simulink model "Horizontal_Turn_Symmetric_DOP"  (Simulink 9.2)
settings: Solver=ode4  StartTime=0.0  StopTime=50  FixedStep=0.01  RelTol=1e-1
values from neighbouring files (symbols this model uses):
  alpha_ = atan(y(3)/y(1))    [Trim_sym.m]    (also in Trim_sym.mat = 0.357010867724)
  b = 2.8956    [Constants_sym.m]    (also in Trim_sym_main.m)
  cbar = 0.18994    [Constants_sym.m]    (also in Trim_sym_main.m)
  Cprop = 1    [Constants_sym.m]    (also in Trim_sym_main.m)
  d2r = pi/180    (= 0.0174532925199)    [Constants_sym.m]    (also in Trim_sym.m; Trim_sym_main.m)
  g = 9.81    [Constants_sym.m]    (also in Trim_sym_main.m)
  Ixx = 0.8244    [Constants_sym.m]    (also in Trim_sym_main.m)
  Ixz = 0.1204    [Constants_sym.m]    (also in Trim_sym_main.m)
  Iyy = 1.135    [Constants_sym.m]    (also in Trim_sym_main.m)
  Izz = 1.759    [Constants_sym.m]    (also in Trim_sym_main.m)
  Kmotor = 80    [Constants_sym.m]    (also in Trim_sym_main.m)
  m = 13.5    [Constants_sym.m]    (also in Trim_sym_main.m)
  q = 0    [Trim_sym.m]
  qbar = 0.5*rho*V^2    [Constants_sym.m]    (also in Trim_sym_main.m = 186.625322459)
  r = 0    [Trim_sym.m]
  r2d = 180/pi    (= 57.2957795131)    [Constants_sym.m]    (also in Trim_sym.m; Trim_sym_main.m)
  rho = p_atm/(287*T_atm)    [Constants_sym.m]    (also in Trim_sym_main.m = 1.44533597728)
  S = 0.55    [Constants_sym.m]    (also in Trim_sym_main.m)
  Sprop = 0.2027    [Constants_sym.m]    (also in Trim_sym_main.m)
  V = 16.07    [Trim_sym.mat]    (also in Trim_sym_main.m)
undefined symbols (not defined in the file or in its folder): F, Light, MIL, sigbuilder_block
libraries: simulink x4, aerolibwind2 x3, sharedtransform x1
(part 2 of 2)

== matlab function EOM/Aerodynamic Constants 2 ==
  data: alpha_ input double; Cx output double; beta_ input double; P input double; Q input double; R input double; delA input double; delE input double; delR input double; Cy output double; Cz output double; Cl output double; Cm output double; Cn output double; u input double; v input double; w input double; CD output double; CL output double
function [Cx,Cy,Cz,Cl,Cm,Cn,CD, CL] = Constants(alpha_,beta_,P,Q,R,delA,delE,delR,u,v,w)

d2r = pi/180;
r2d = 180/pi;

%% CONSTANTS
% Geometric / mass properties data
g = 9.81; 
ALT = 1000; % altitude (in m)
V = sqrt(u^2 + v^2 + w^2); % velocity (in m/s)

% max_thrust = 32000*g/2.2046;
if (ALT <= 11000) 
   T_atm = 288.15-0.0065*ALT; % atmospheric temp.(in Kelvin)
   p_atm = 101325*(T_atm/288.15)^(9.81/(287*0.0065));  % atmospheric pressure (pascal)
else 
   T_atm = 216.65;
   p_atm = 22632*exp(-9.81*(ALT-11000)/(287*216.65)); 
end   
R1 = 287.1;  % Gas constant (m2/s2/K)
ss = sqrt(1.4*R1*T_atm); % sound velocity (m/s)
M = V/ss;
rho = p_atm/(287*T_atm);
rho_sl = 1.225; % density @ sea-level (kg/m3)
% T = max_thrust * (rho / rho_sl)^0.7 * (1 - exp((ALT - 17000) / 2000));
% T = 0.9*max_thrust*(0.88+0.24*(abs(M-0.6))^1.4)*(rho/rho_sl)^0.8;

lz = 0;
lx = 0;
 m = 13.5;
 W = m*g;
 S = 0.55;
 qbar = 0.5*rho*V^2;
 cbar = 0.18994;
b = 2.8956; % ft -> m  
 Ixx = 0.8244; % slugs ft2 -> Kg m2
Iyy = 1.135;
Izz = 1.759;
Ixz = 0.1204;

%%

CD0 = 0.03;
CDalpha = 0.30;
CDQ=0;
CDdeltae=0;
CDP=0.0437;
CD = (CD0+CDalpha*alpha_+(CDQ*cbar*Q/(2*V))+CDdeltae*delE+(CDP*b*P/(2*V)));
 
CY0=0;
CYbeta = -0.98;
CYP = 0;
CYR = 0;
CYdeltaa = 0;
CYdeltar = -0.17;

CY = (CY0+CYbeta*beta_+(CYP*b*P/(2*V))+(CYR*b*R/(2*V))+CYdeltaa*delA+CYdeltar*delR);
 
CL0=0.28;
CLalpha = 3.45;
CLQ=0;
CLdeltae = -0.36;
CL = (CL0 + CLalpha*alpha_+CLdeltae*delE+(CLQ*cbar*Q/(2*V)));
 
CM0 = -0.02338;
CMalpha = -0.38;
CMQ = -3.6;
CMdeltae = -0.5;
Cm = (CM0+CMalpha*alpha_+CMdeltae*delE+(CMQ*cbar*Q/(2*V)));
 
Cl0=0;
Clbeta =-0.12;
ClP = -0.26;
ClR = 0.14;
Cldeltaa = 0.08;
Cldeltar = 0.105;

Cl = (Cl0+Clbeta*beta_+(ClP*b*P/(2*V))+(ClR*b*R/(2*V))+Cldeltaa*delA+ Cldeltar*delR);
 
Cn0=0;
Cnbeta = 0.25;
CnP = 0.022;
CnR = -0.35;
Cndeltaa = 0.06;
Cndeltar = -0.032;
Cn = (Cn0+Cnbeta*beta_+(CnP*b*P/(2*V))+(CnR*b*R/(2*V))+Cndeltaa*delA+Cndeltar*delR);
 
Cx = (-CD*cos(alpha_)*cos(beta_)-CY*cos(alpha_)*sin(beta_)+CL*sin(alpha_));
Cy = (CY*cos(beta_)-CD*sin(beta_));
Cz = (-CD*sin(alpha_)*cos(beta_)-CY*sin(alpha_)*sin(beta_)-CL*cos(alpha_));

== matlab function Lateral Directional Controller (backstepping)/Back_Step ==
  data: alpha_ input double; M1 output double; beta_ input double; p_ input double; r_ input double; phi input double; V input double; phi_ref input double; phi_ref_dot input double; beta_ref input double; beta_ref_dot input double; p_ref_dot input double; r_ref_dot input double
function M1 = Back_Step(alpha_,beta_,p_,r_,phi,V, phi_ref,phi_ref_dot,beta_ref,beta_ref_dot, p_ref_dot,r_ref_dot)

M1=zeros(4,1);
x1 = [phi;beta_];
x1d = [phi_ref;beta_ref];
x1d_dot	 = [phi_ref_dot;beta_ref_dot];

x2 = [p_;r_];
x2d_dot = [p_ref_dot;r_ref_dot];


%%
d2r = pi/180;
r2d = 180/pi;

%% CONSTANTS
% Geometric / mass properties data
g = 9.81; 
ALT =1000;
% H = 3000; % altitude (in m)
% V = sqrt(u^2 + v^2 + w^2); % velocity (in m/s)
max_thrust = 22;
if (ALT <= 11000) 
   T_atm = 288.15-0.0065*ALT; % atmospheric temp.(in Kelvin)
   p_atm = 101325*(T_atm/288.15)^(9.81/(287*0.0065));  % atmospheric pressure (pascal)
else 
   T_atm = 216.65;
   p_atm = 22632*exp(-9.81*(ALT-11000)/(287*216.65)); 
end   
R1 = 287.1;  % Gas constant (m2/s2/K)
ss = sqrt(1.4*R1*T_atm); % sound velocity (m/s)
 M = V/ss;

rho = p_atm/(287*T_atm);
% rho=1.2682;
rho_sl = 1.225; % density @ sea-level (kg/m3)

% T = max_thrust * (rho / rho_sl)^0.7 * (1 - exp((ALT - 17000) / 2000));
% T = 0.9*max_thrust*(0.88+0.24*(abs(M-0.6))^1.4)*(rho/rho_sl)^0.8;

 m = 13.5;
 W = m*g;
 S = 0.55;
 qbar = 0.5*rho*V^2;
 cbar = 0.18994;
b = 2.8956; % ft -> m  
 Ixx = 0.8244; % slugs ft2 -> Kg m2
Iyy = 1.135;
Izz = 1.759;
Ixz = 0.1204;




%%
%  CD0 = 0.03;
%  CDalpha = 0.30;
%  CDQ=0;
%  CDdeltae=0;
% CDP=0.0437;
%  CD = (CD0+CDalpha*alpha_+(CDQ*cbar*Q/(2*V))+CDdeltae*delE+(CDP*b*P/(2*V)));
%  
%  CY0=0;
 CYbeta = -0.98;
%  CYP = 0;
%  CYR = 0;
%  CYdeltaa = 0;
% CYdeltar = -0.17;
% 
%  CY = (CY0+CYbeta*beta_+(CYP*b*P/(2*V))+(CYR*b*R/(2*V))+CYdeltaa*delA+CYdeltar*delR);
%  
% CL0=0.28;
% CLalpha = 3.45;
% CLQ=0;
% CLdeltae = -0.36;
%  CL = (CL0 + CLalpha*alpha_+CLdeltae*delE+(CLQ*cbar*Q/(2*V)));
%  
% CM0 = -0.02338;
%  CMalpha = -0.38;
%  CMQ = -3.6;
%  CMdeltae = -0.5;
%  Cm = (CM0+CMalpha*alpha_+CMdeltae*delE+(CMQ*cbar*Q/(2*V)));
 
 Cl0=0;
 Clbeta =-0.12;
 ClP = -0.26;
 ClR = 0.14;
%  Cldeltaa = 0.08;
% Cldeltar = 0.105;

%   Cl = (Cl0+Clbeta*beta_+(ClP*b*P/(2*V))+(ClR*b*R/(2*V))+Cldeltaa*delA+ Cldeltar*delR);
 
 Cn0=0;
  Cnbeta = 0.25;
 CnP = 0.022;
 CnR = -0.35;
% Cndeltaa = 0.06;
% Cndeltar = -0.032;
%   Cn = (Cn0+Cnbeta*beta_+(CnP*b*P/(2*V))+(CnR*b*R/(2*V))+Cndeltaa*delA+Cndeltar*delR);
  
  
Cl_state =  (Cl0+Clbeta*beta_+(ClP*b*p_/(2*V))+(ClR*b*r_/(2*V)));
Cn_state =  (Cn0+Cnbeta*beta_+(CnP*b*p_/(2*V))+(CnR*b*r_/(2*V)));
 
 %% controller calculation

 %% controller calculation

f1 = [0;
      (g/V)*sin(phi)*cos(alpha_)+(0.5*rho*V^2*S*CYbeta*beta_)/(m*V);];
      
f2 = [1, alpha_*cos(phi);
       alpha_ , -1];

c =   Ixx*Izz - Ixz^2 ;
c3=   Izz/c;
c4=  Ixz/c;
c9=  Ixx/c;

I = [c3,c4;
       c4 , c9;];

f3 = I*[qbar*S*b*Cl_state;qbar*S*b*Cn_state];
% f3 = [c3*qbar*S*b*Cl_state;c9*qbar*S*b*Cn_state];
    
l1 = [15 10];
K1 = diag(l1);
    
l2 = [10 5];
K2 = diag(l2);  
K11 = 0.1;
K22 = 0.1;

E1 = (x1-x1d);
N1 = integral1(E1,0,15);

 
x2d = (inv(f2))*(- K1*(x1-x1d)-((K11^2)*N1) + x1d_dot-f1);

E2 = (x2-x2d);
N2 = integral2(E2,0,15);

U1 = -K2*(x2 - x2d) -f3 + x2d_dot - (f2'*(x1-x1d))-(N2*(K22^2));

M1=[U1;x2d];

% MXc = U(1);
% MYc = U(2);
% MZc = U(3);
% 
% p_ref = x2d(1);
% q_ref = x2d(2);
% r_ref = x2d(3);

== matlab function Subsystem/Throttle controller ==
  data: alpha_ input double; Ft output double; gama_ input double; V input double; Vref input double; Vref_dot input double; P input double; Q input double; velocity_error input double
function Ft = fcn(alpha_, gama_, V, Vref, Vref_dot, P, Q, velocity_error)

m = 13.500;
g = 9.8100;
b = 2.89560;
cbar = 0.189940;
ALT = 1000;

if (ALT <= 11000) 
   T_atm = 288.15-0.0065*ALT; % atmospheric temp.(in Kelvin)
   p_atm = 101325*(T_atm/288.15)^(9.81/(287*0.0065));  % atmospheric pressure (pascal)
else 
   T_atm = 216.65;
   p_atm = 22632*exp(-9.81*(ALT-11000)/(287*216.65)); 
end   
R1 = 287.1;  % Gas constant (m2/s2/K)
ss = sqrt(1.4*R1*T_atm); % sound velocity (m/s)
M = V/ss;

rho = p_atm/(287*T_atm);

%rho = 1.11177716839116;
S = 0.550;

Kv = 12.6;
Kvv = 5.5;

CD0 = 0.03;
CDalpha = 0.30;
CDQ=0;
CDdeltae=0;
CDP=0.0437;
CD = CD0+CDalpha*alpha_+(CDQ*cbar*Q/(2*V))+(CDP*b*P/(2*V));
%Cd = Cd0 + k1*alpha + k2*alpha*alpha;
%Vref^2 + (V-Vref)^2

Ft = (m/cos(alpha_))*(g*sin(gama_) - Kv*(V - Vref) - Kvv*velocity_error + Vref_dot + 0.5*rho*(V^2)*(S/m)*CD);

== matlab function Longitudinal Controller (backstepping) ==
  data: theta_ref input double; theta_ref_d input double; q_ref output double; theta input double; phi input double; q input double; p input double; r input double; q_ref_d input double; alpha input double; alpha_d input double; delta_e output double; V input double
function [q_ref, delta_e] = fcn(theta_ref, theta_ref_d, theta, phi, q, p, r, q_ref_d, alpha, alpha_d, V)

%% CONSTANTS
% Geometric / mass properties data
g = 9.81; 
ALT =1000;
% H = 3000; % altitude (in m)
% V = sqrt(u^2 + v^2 + w^2); % velocity (in m/s)
max_thrust = 22;
if (ALT <= 11000) 
   T_atm = 288.15-0.0065*ALT; % atmospheric temp.(in Kelvin)
   p_atm = 101325*(T_atm/288.15)^(9.81/(287*0.0065));  % atmospheric pressure (pascal)
else 
   T_atm = 216.65;
   p_atm = 22632*exp(-9.81*(ALT-11000)/(287*216.65)); 
end   
R1 = 287.1;  % Gas constant (m2/s2/K)
ss = sqrt(1.4*R1*T_atm); % sound velocity (m/s)
 M = V/ss;

rho = p_atm/(287*T_atm);
% rho=1.2682;
rho_sl = 1.225; % density @ sea-level (kg/m3)

% T = max_thrust * (rho / rho_sl)^0.7 * (1 - exp((ALT - 17000) / 2000));
% T = 0.9*max_thrust*(0.88+0.24*(abs(M-0.6))^1.4)*(rho/rho_sl)^0.8;

 m = 13.5;
 W = m*g;
 S = 0.55;
 qbar = 0.5*rho*V^2;
 cbar = 0.18994;
b = 2.8956; % ft -> m  
 Ixx = 0.8244; % slugs ft2 -> Kg m2
Iyy = 1.135;
Izz = 1.759;
Ixz = 0.1204;




%%
%  CD0 = 0.03;
%  CDalpha = 0.30;
%  CDQ=0;
%  CDdeltae=0;
% CDP=0.0437;
%  CD = (CD0+CDalpha*alpha_+(CDQ*cbar*Q/(2*V))+CDdeltae*delE+(CDP*b*P/(2*V)));
%  
%  CY0=0;
 CYbeta = -0.98;
%  CYP = 0;
%  CYR = 0;
%  CYdeltaa = 0;
% CYdeltar = -0.17;
% 
%  CY = (CY0+CYbeta*beta_+(CYP*b*P/(2*V))+(CYR*b*R/(2*V))+CYdeltaa*delA+CYdeltar*delR);
%  
% CL0=0.28;
% CLalpha = 3.45;
% CLQ=0;
% CLdeltae = -0.36;
%  CL = (CL0 + CLalpha*alpha_+CLdeltae*delE+(CLQ*cbar*Q/(2*V)));
%  
CM0 = -0.02338;
CMalpha = -0.38;
CMQ = -3.6;
CMalphadot = -10.4;
CMdeltae = -0.5;
Cm = (CM0+CMalpha*alpha+(CMQ*q+CMalphadot*alpha_d)*cbar/(2*V));
 
 %Cl0=0;
% Clbeta =-0.12;
 %ClP = -0.26;
% ClR = 0.14;
%  Cldeltaa = 0.08;
% Cldeltar = 0.105;

%   Cl = (Cl0+Clbeta*beta_+(ClP*b*P/(2*V))+(ClR*b*R/(2*V))+Cldeltaa*delA+ Cldeltar*delR);
 
 %Cn0=0;
% Cnbeta = 0.25;
 %CnP = 0.022;
 %CnR = -0.35;
% Cndeltaa = 0.06;
% Cndeltar = -0.032;
%   Cn = (Cn0+Cnbeta*beta_+(CnP*b*P/(2*V))+(CnR*b*R/(2*V))+Cndeltaa*delA+Cndeltar*delR);
  
  
%Cl_state =  (Cl0+Clbeta*beta_+(ClP*b*p_/(2*V))+(ClR*b*r_/(2*V)));
%Cn_state =  (Cn0+Cnbeta*beta_+(CnP*b*p_/(2*V))+(CnR*b*r_/(2*V)));

%Controller calculations

Kq =4;
Ktheta = 4;

q_ref = (Ktheta*(theta_ref - theta) + r*sin(phi) + theta_ref_d)/cos(phi);
%q_ref = Ktheta*(theta_ref - theta)+ theta_ref_d;
delta_e = (Iyy/(rho*S*cbar*CMdeltae))*((theta_ref - theta)*cos(phi) - Kq*(q - q_ref) + ((Ixx - Izz)/Iyy)*p*r + (Ixz/Iyy)*(p^2 - r^2) + q_ref_d - (rho*S*cbar/Iyy)*Cm );
%delta_e = (theta_ref - theta) - Kq*(q - q_ref) + q_ref_d - (rho*S*cbar/Iyy)*Cm ;

== matlab function EOM/MATLAB Function ==
  data: V input double; V_dot output double; alpha_dot output double; beta_dot output double; Ft input double; alpha_ input double; beta_ input double; gama input double; gama_dot output double; Cl input double; Fx input double; Fy input double; Fz input double
function [V_dot, alpha_dot, beta_dot, gama_dot]= fcn(V, Ft, alpha_, beta_, gama, Cl, Fx, Fy, Fz)
m = 13.5;
g = 9.81;
rho = 1.11177716839116;
S = 0.55000;
L = 0.5*rho*V*V*S*Cl;
Cd0 = 0.05;
k1 = 0.05;
k2 = 0.05;
Cd = Cd0 + k1*alpha_ + k2*alpha_*alpha_;
D = 0.5*rho*V*V*S*Cd;
V_dot = -g*sin(gama)+1/m*Fx;
gama_dot = (1/m*V)*(L + Ft*sin(alpha_) - m*g*cos(gama));
alpha_dot = q - p*cos(alpha_)*tan(beta_) - r*sin(alpha_)*tan(beta_) + (g/V)*sec(beta_)*cos;
beta_dot = ;

== matlab function Subsystem1/Flight Path angle controller ==
  data: V input double; delE output double; theta input double; gama_ref input double; gama_ input double; q input double; gamma_error input double
function delE = fcn(V, theta, gama_ref, gama_, q, gamma_error)
rho = 1.11177716839116;
S = 0.550;
cbar = 0.189940;
Iyy = 1.1350;
alpha_trim = 0.357010867723814;

Cm_delE = -0.5;
Cm0 = -0.02338;
Cm_alpha = -0.38;
Cm_q = -3.6;

K1 = 0.2;
K2 = 5;
K3 = 50;
Ki = 0.5;

b_2 = 0.5*rho*V*V*S*cbar/Iyy;
b_delE = 0.5*rho*V*V*S*cbar*Cm_delE/Iyy;

delE = (1/b_delE)*(-K3*(q + K2*(theta - gama_ref - alpha_trim + K1*(gama_ - gama_ref)+ Ki*gamma_error)) - b_2*(Cm0 + Cm_alpha*(theta - gama_) + Cm_q*cbar*q/(2*V)));

== matlab function EOM/MATLAB Function1 ==
  data: alpha input double; Fx output double; beta input double; V input double; Cx input double; Cy input double; Cz input double; Tx input double; Ty input double; Tz input double; Fy output double; Fz output double
function [Fx, Fy, Fz]= fcn(alpha, beta, V, Cx, Cy, Cz, Tx, Ty, Tz)

rho = 1.11177716839116;

qbar = 0.5*rho*V*V;
[Fx Fy Fz]' = [cos(alpha)*cos(beta) sin(beta) sin(alpha)*cos(beta); -cos(alpha)*sin(beta) cos(beta) -sin(alpha)*sin*(beta); -sin(alpha) 0 cos(alpha)] * [qbar*S*Cx + Tx;qbar*S*Cy + Ty; qbar*S*Cz + Tz] ;
